simulink model "Online_Ordering_System_Component_Architecture"  (R2025a)
settings: Solver=VariableStepDiscrete  StartTime=0.0  StopTime=10.0  MaxStep=1  RelTol=1e-3
(part 2 of 2)

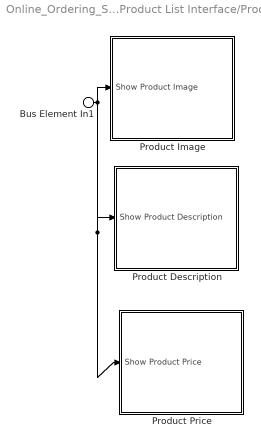
== system Online_Ordering_System_Component_Architecture/Ordering System/Product List Interface/Product Menu Interface ==
  Bus Element In1 : Inport  PortName=Show Product Information
  Product Description : Subsystem
      settings: PortSchema="{\"entries\":[{\"content\":{\"headerSize\":26,\"margin\":15,\"minimumSpacing\":25,\"sides\":[{\"content\":{\"connectorIds\":[\"In1\"]},\"type\":\"ConnectorPlacement.EquallySpacedRectSide\",\"uuid\":\"d2ebed04-42f4-4bd6-aa56-c214d37abe86\"},{\"content\":{\"side\":\"RIGHT\"},\"type\":\"ConnectorPlacement.EquallySpacedRectSide\",\"uuid\":\"0a328130-2da5-4535-b8fd-dee261bd04a3\"},{\"content\":{\"side\":\"TOP\"},\"type\":\"ConnectorPlacement.EquallySpacedRectSide\",\"uuid\":\"410ea5eb-e20b-4523-bb7e-a86253749ceb\"}]},\"type\":\"ConnectorPlacement.EquallySpacedConnector\",\"uuid\":\"5600d62f-d466-4629-981b-50f24b9b11a3\"}],\"packageUris\":[\"http://schema.mathworks.com/mf0/Connector/R2020b\"],\"version\":\"1.0\"}"
  Product Image : Subsystem
      settings: PortSchema="{\"entries\":[{\"content\":{\"headerSize\":26,\"margin\":15,\"minimumSpacing\":25,\"sides\":[{\"content\":{\"connectorIds\":[\"In1\"]},\"type\":\"ConnectorPlacement.EquallySpacedRectSide\",\"uuid\":\"d2ebed04-42f4-4bd6-aa56-c214d37abe86\"},{\"content\":{\"side\":\"RIGHT\"},\"type\":\"ConnectorPlacement.EquallySpacedRectSide\",\"uuid\":\"0a328130-2da5-4535-b8fd-dee261bd04a3\"},{\"content\":{\"side\":\"TOP\"},\"type\":\"ConnectorPlacement.EquallySpacedRectSide\",\"uuid\":\"410ea5eb-e20b-4523-bb7e-a86253749ceb\"}]},\"type\":\"ConnectorPlacement.EquallySpacedConnector\",\"uuid\":\"5600d62f-d466-4629-981b-50f24b9b11a3\"}],\"packageUris\":[\"http://schema.mathworks.com/mf0/Connector/R2020b\"],\"version\":\"1.0\"}"
  Product Price : Subsystem
      settings: PortSchema="{\"entries\":[{\"content\":{\"headerSize\":26,\"margin\":15,\"minimumSpacing\":25,\"sides\":[{\"content\":{\"connectorIds\":[\"In1\"]},\"type\":\"ConnectorPlacement.EquallySpacedRectSide\",\"uuid\":\"d2ebed04-42f4-4bd6-aa56-c214d37abe86\"},{\"content\":{\"side\":\"RIGHT\"},\"type\":\"ConnectorPlacement.EquallySpacedRectSide\",\"uuid\":\"0a328130-2da5-4535-b8fd-dee261bd04a3\"},{\"content\":{\"side\":\"TOP\"},\"type\":\"ConnectorPlacement.EquallySpacedRectSide\",\"uuid\":\"410ea5eb-e20b-4523-bb7e-a86253749ceb\"}]},\"type\":\"ConnectorPlacement.EquallySpacedConnector\",\"uuid\":\"5600d62f-d466-4629-981b-50f24b9b11a3\"}],\"packageUris\":[\"http://schema.mathworks.com/mf0/Connector/R2020b\"],\"version\":\"1.0\"}"
  wires:
  Bus Element In1/1 -> Product Price/1(Show Product Price), Product Description/1(Show Product Description), Product Image/1(Show Product Image)

== system Online_Ordering_System_Component_Architecture/Product Management System/Product Information/Menu Interface ==
  Bus Element In1 : Inport  PortName=Product Information Edit
  Bus Element Out1 : Outport  PortName=Edit Product Detail

== system Online_Ordering_System_Component_Architecture/Product Management System/Product Information/Product Description Interface ==
  Bus Element In1 : Inport  PortName=Edit Description

== system Online_Ordering_System_Component_Architecture/Product Management System/Product Information/Product Images Interface ==
  Bus Element In1 : Inport  PortName=Edit Image

== system Online_Ordering_System_Component_Architecture/Product Management System/Product Information/Product Price Interface ==
  Bus Element In1 : Inport  PortName=Edit Price

== system Online_Ordering_System_Component_Architecture/Ordering System/Product List Interface/Product Menu Interface/Product Description ==
  Bus Element In1 : Inport  PortName=Show Product Description

== system Online_Ordering_System_Component_Architecture/Ordering System/Product List Interface/Product Menu Interface/Product Image ==
  Bus Element In1 : Inport  PortName=Show Product Image

== system Online_Ordering_System_Component_Architecture/Ordering System/Product List Interface/Product Menu Interface/Product Price ==
  Bus Element In1 : Inport  PortName=Show Product Price
